simulink model "experiment_toplevel"  (R2016a)
settings: Solver=ode15s  StartTime=0.0  StopTime=20  MaxStep=1e-2  RelTol=1e-4
PreLoadFcn:
  | minitaurParameters
values from neighbouring files (symbols this model uses):
  angular_ctrl_d = 1    [minitaurParameters.m]
  angular_ctrl_i = 1    [minitaurParameters.m]
  angular_ctrl_p = 100    [minitaurParameters.m]
  enc_zero_IA = -1.25*pi    (= -3.92699081699)    [minitaurParameters.m]
  enc_zero_IB = -0.25*pi    (= -0.785398163397)    [minitaurParameters.m]
  enc_zero_IIA = 1.25*pi    (= 3.92699081699)    [minitaurParameters.m]
  enc_zero_IIB = 1.25*pi    (= 3.92699081699)    [minitaurParameters.m]
  enc_zero_IIIA = 0.5*pi    (= 1.57079632679)    [minitaurParameters.m]
  enc_zero_IIIB = 1.5*pi    (= 4.71238898038)    [minitaurParameters.m]
  enc_zero_IVA = -0.25*pi    (= -0.785398163397)    [minitaurParameters.m]
  enc_zero_IVB = 0.5*pi    (= 1.57079632679)    [minitaurParameters.m]
  fore_lag = fore_lag_vals(j)    [experiment1.m]    (also in experiment1_parfor_accelerator.m = 0; minitaurParameters.m = 0.45)
  ground_frame_depth = 0.5    [minitaurParameters.m]
  ground_length = 100    [minitaurParameters.m]
  ground_width = 10    [minitaurParameters.m]
  init_theta_IA = -pi/4    (= -0.785398163397)    [minitaurParameters.m]
  init_theta_IB = pi/4    (= 0.785398163397)    [minitaurParameters.m]
  init_theta_IIA = -pi/4    (= -0.785398163397)    [minitaurParameters.m]
  init_theta_IIB = pi/4    (= 0.785398163397)    [minitaurParameters.m]
  init_theta_IIIA = -pi/4    (= -0.785398163397)    [minitaurParameters.m]
  init_theta_IIIB = pi/4    (= 0.785398163397)    [minitaurParameters.m]
  init_theta_IVA = -pi/4    (= -0.785398163397)    [minitaurParameters.m]
  init_theta_IVB = pi/4    (= 0.785398163397)    [minitaurParameters.m]
  l1 = 100e-3    (= 0.1)    [minitaurParameters.m]
  l2 = 200e-3    (= 0.2)    [minitaurParameters.m]
  leg_joint_radius = 3e-3    (= 0.003)    [minitaurParameters.m]
  lr_sync = 1    [experiment1.m]    (also in experiment1_parfor_accelerator.m; minitaurParameters.m = 0)
  model = 'experiment_toplevel'    [experiment1_parfor_accelerator.m]
  period = period_vals(i)    [experiment1.m]    (also in experiment1_parfor_accelerator.m = 1.5; minitaurParameters.m = 0.33)
  phi_0 = 0.5*asin(l1/l2)    [experiment1.m]    (also in experiment1_parfor_accelerator.m; minitaurParameters.m)
  r_0 = l2    [experiment1.m]    (also in experiment1_parfor_accelerator.m; minitaurParameters.m = 0.2)
  r_x = 0.3*l1    [experiment1.m]    (also in experiment1_parfor_accelerator.m = 0.5*l1; minitaurParameters.m = 0.05)
  r_y = 0.2*l1    [experiment1.m]    (also in experiment1_parfor_accelerator.m = 0.3*l1; minitaurParameters.m = 0.03)
  radial_ctrl_d = 1    [minitaurParameters.m]
  radial_ctrl_i = 1    [minitaurParameters.m]
  radial_ctrl_p = 80    [minitaurParameters.m]
  safety_limit = 10e-3    (= 0.01)    [minitaurParameters.m]
undefined symbols (not defined in the file or in its folder): Axis, Fn, minitaurParams, r_stance, r_swing, stance_frac, X, Y, Z
undefined symbols (not defined in the file): leg_joint_fric_bw, leg_joint_mu_k, leg_joint_mu_s, leg_joint_vel_thresh, motor_kt, motor_kv, motor_r, motor_torque_sat
libraries: sm_lib x453, fl_lib x132, nesl_utility x31, Contact_Forces_Lib x28, simulink x19
(part 3 of 13)

== system experiment_toplevel/GR Minitaur/minitaur_leg_linkages_III ==
  Joint Friction Model : Subsystem  Variant=on  OverrideUsingVariant=stick-slip  mask(Joint Friction Model){modelVariant=Stick-Slip Friction, leg_joint_radius=leg_joint_radius, linear_region_thresh=leg_joint_vel_thresh, mu_k=leg_joint_mu_k, mu_s=leg_joint_mu_s, fric_bandwidth=leg_joint_fric_bw, mu_brk=0, fric_visc_coeff=0, trans_coeff=0}
      mask prompts: modelVariant "Friction Model"; leg_joint_radius "Leg Joint Effective Radius [m]"; linear_region_thresh "Linear Region Velocity Threshold [m/s]"; mu_k "Kinetic Friction Coefficient []"; mu_s "Static Friction Coefficient []"; fric_bandwidth "Friction Model Bandwidth [Hz]"; mu_brk "Breakaway Friction Coefficient []"; fric_visc_coeff "Viscous Friction Coefficient [N*s/m]"; trans_coeff "Transition Approximation Coefficient [s/m]"
      mask help: Models rotational friction present in passive joints. Two options available: stick-slip, and an advanced model that includes viscous and Stribeck friction. Note that in all models, friction is calculated as translational force couple, which is then converted to a friction torque (multiplied by effective joint diameter).
      mask TypeOptions modelVariant: Full Friction | Stick-Slip Friction
      mask Callback modelVariant:
      | currVariant = get_param(gcb,'modelVariant')
      | 
      | switch currVariant
      |     case 'Stick-Slip Friction'
      |         set_param(gcb,'OverrideUsingVariant','stick-slip')
      |         set_param(gcb,'MaskVisibilities',{'on';'on';'on';'on';'on';'on';'off';'off';'off'})
      |     case 'Full Friction'
      |         set_param(gcb,'OverrideUsingVariant','full')
      |         set_param(gcb,'MaskVisibilities',{'on';'on';'on';'on';'off';'off';'on';'on';'on'})
      | 
      | end
  Joint Friction Model1 : Subsystem  Variant=on  OverrideUsingVariant=stick-slip  mask(Joint Friction Model){modelVariant=Stick-Slip Friction, leg_joint_radius=leg_joint_radius, linear_region_thresh=leg_joint_vel_thresh, mu_k=leg_joint_mu_k, mu_s=leg_joint_mu_s, fric_bandwidth=leg_joint_fric_bw, mu_brk=0, fric_visc_coeff=0, trans_coeff=0}
      mask prompts: modelVariant "Friction Model"; leg_joint_radius "Leg Joint Effective Radius [m]"; linear_region_thresh "Linear Region Velocity Threshold [m/s]"; mu_k "Kinetic Friction Coefficient []"; mu_s "Static Friction Coefficient []"; fric_bandwidth "Friction Model Bandwidth [Hz]"; mu_brk "Breakaway Friction Coefficient []"; fric_visc_coeff "Viscous Friction Coefficient [N*s/m]"; trans_coeff "Transition Approximation Coefficient [s/m]"
      mask help: Models rotational friction present in passive joints. Two options available: stick-slip, and an advanced model that includes viscous and Stribeck friction. Note that in all models, friction is calculated as translational force couple, which is then converted to a friction torque (multiplied by effective joint diameter).
      mask TypeOptions modelVariant: Full Friction | Stick-Slip Friction
      mask Callback modelVariant:
      | currVariant = get_param(gcb,'modelVariant')
      | 
      | switch currVariant
      |     case 'Stick-Slip Friction'
      |         set_param(gcb,'OverrideUsingVariant','stick-slip')
      |         set_param(gcb,'MaskVisibilities',{'on';'on';'on';'on';'on';'on';'off';'off';'off'})
      |     case 'Full Friction'
      |         set_param(gcb,'OverrideUsingVariant','full')
      |         set_param(gcb,'MaskVisibilities',{'on';'on';'on';'on';'off';'off';'on';'on';'on'})
      | 
      | end
  Joint Friction Model2 : Subsystem  Variant=on  OverrideUsingVariant=stick-slip  mask(Joint Friction Model){modelVariant=Stick-Slip Friction, leg_joint_radius=leg_joint_radius, linear_region_thresh=leg_joint_vel_thresh, mu_k=leg_joint_mu_k, mu_s=leg_joint_mu_s, fric_bandwidth=leg_joint_fric_bw, mu_brk=0, fric_visc_coeff=0, trans_coeff=0}
      mask prompts: modelVariant "Friction Model"; leg_joint_radius "Leg Joint Effective Radius [m]"; linear_region_thresh "Linear Region Velocity Threshold [m/s]"; mu_k "Kinetic Friction Coefficient []"; mu_s "Static Friction Coefficient []"; fric_bandwidth "Friction Model Bandwidth [Hz]"; mu_brk "Breakaway Friction Coefficient []"; fric_visc_coeff "Viscous Friction Coefficient [N*s/m]"; trans_coeff "Transition Approximation Coefficient [s/m]"
      mask help: Models rotational friction present in passive joints. Two options available: stick-slip, and an advanced model that includes viscous and Stribeck friction. Note that in all models, friction is calculated as translational force couple, which is then converted to a friction torque (multiplied by effective joint diameter).
      mask TypeOptions modelVariant: Full Friction | Stick-Slip Friction
      mask Callback modelVariant:
      | currVariant = get_param(gcb,'modelVariant')
      | 
      | switch currVariant
      |     case 'Stick-Slip Friction'
      |         set_param(gcb,'OverrideUsingVariant','stick-slip')
      |         set_param(gcb,'MaskVisibilities',{'on';'on';'on';'on';'on';'on';'off';'off';'off'})
      |     case 'Full Friction'
      |         set_param(gcb,'OverrideUsingVariant','full')
      |         set_param(gcb,'MaskVisibilities',{'on';'on';'on';'on';'off';'off';'on';'on';'on'})
      | 
      | end
  ReferenceFrame : sm_lib/Frames and Transforms/Reference Frame
  Revolute : sm_lib/Joints/Revolute Joint  SenseConstraintForce=off  SenseConstraintForceX=off  SenseConstraintForceY=off  SenseConstraintForceZ=off  SenseConstraintTorque=off  SenseConstraintTorqueX=off  SenseConstraintTorqueY=off  SenseConstraintTorqueZ=off  SenseTotalForce=on  SenseTotalForceX=off  SenseTotalForceY=off  SenseTotalForceZ=off  SenseTotalTorque=off  SenseTotalTorqueX=off  SenseTotalTorqueY=off  SenseTotalTorqueZ=off  CompositeWrenchDir=FollowerOnBase  CompositeWrenchFrame=BaseFrame  EquilibriumPosition=0  EquilibriumPositionUnits=rad  SpringStiffness=0  SpringStiffnessUnits=m*N/rad  DampingCoefficient=0  DampingCoefficientUnits=m*s*N/rad  TorqueActuationMode=InputTorque  MotionActuationMode=ComputedMotion  SensePosition=off  SenseVelocity=on  SenseAcceleration=off  SenseTorqueForce=off  PositionTargetSpecify=off  PositionTargetPriority=Low  PositionTargetValue=minitaurParams.RevoluteJoint(1).Rz.Pos  PositionTargetValueUnits=deg  VelocityTargetSpecify=off  VelocityTargetPriority=High  VelocityTargetValue=0  VelocityTargetValueUnits=deg/s
  Revolute1 : sm_lib/Joints/Revolute Joint  SenseConstraintForce=off  SenseConstraintForceX=off  SenseConstraintForceY=off  SenseConstraintForceZ=off  SenseConstraintTorque=off  SenseConstraintTorqueX=off  SenseConstraintTorqueY=off  SenseConstraintTorqueZ=off  SenseTotalForce=on  SenseTotalForceX=off  SenseTotalForceY=off  SenseTotalForceZ=off  SenseTotalTorque=off  SenseTotalTorqueX=off  SenseTotalTorqueY=off  SenseTotalTorqueZ=off  CompositeWrenchDir=FollowerOnBase  CompositeWrenchFrame=BaseFrame  EquilibriumPosition=0  EquilibriumPositionUnits=rad  SpringStiffness=0  SpringStiffnessUnits=m*N/rad  DampingCoefficient=0  DampingCoefficientUnits=m*s*N/rad  TorqueActuationMode=InputTorque  MotionActuationMode=ComputedMotion  SensePosition=off  SenseVelocity=on  SenseAcceleration=off  SenseTorqueForce=off  PositionTargetSpecify=on  PositionTargetPriority=Low  PositionTargetValue=init_toe_joint_l  PositionTargetValueUnits=rad  VelocityTargetSpecify=off  VelocityTargetPriority=High  VelocityTargetValue=0  VelocityTargetValueUnits=deg/s
  Revolute2 : sm_lib/Joints/Revolute Joint  SenseConstraintForce=off  SenseConstraintForceX=off  SenseConstraintForceY=off  SenseConstraintForceZ=off  SenseConstraintTorque=off  SenseConstraintTorqueX=off  SenseConstraintTorqueY=off  SenseConstraintTorqueZ=off  SenseTotalForce=on  SenseTotalForceX=off  SenseTotalForceY=off  SenseTotalForceZ=off  SenseTotalTorque=off  SenseTotalTorqueX=off  SenseTotalTorqueY=off  SenseTotalTorqueZ=off  CompositeWrenchDir=FollowerOnBase  CompositeWrenchFrame=BaseFrame  EquilibriumPosition=0  EquilibriumPositionUnits=rad  SpringStiffness=0  SpringStiffnessUnits=m*N/rad  DampingCoefficient=0  DampingCoefficientUnits=m*s*N/rad  TorqueActuationMode=InputTorque  MotionActuationMode=ComputedMotion  SensePosition=off  SenseVelocity=on  SenseAcceleration=off  SenseTorqueForce=off  PositionTargetSpecify=off  PositionTargetPriority=Low  PositionTargetValue=minitaurParams.RevoluteJoint(3).Rz.Pos  PositionTargetValueUnits=deg  VelocityTargetSpecify=off  VelocityTargetPriority=High  VelocityTargetValue=0  VelocityTargetValueUnits=deg/s
  Transform : sm_lib/Frames and Transforms/Rigid Transform  TranslationMethod=Cartesian  TranslationLengthUnit=mm  TranslationStandardAxis=+Z  TranslationStandardOffset=0  TranslationCartesianOffset=minitaurParams.RigidTransform(16).translation  TranslationROffset=0  TranslationROffsetUnits=m  TranslationZOffset=0  TranslationZOffsetUnits=m  TranslationThetaOffset=0  TranslationThetaOffsetUnits=deg  RotationMethod=ArbitraryAxis  RotationAngleUnits=rad  RotationStandardAxis=+Z  RotationAngle=minitaurParams.RigidTransform(16).angle  RotationArbitraryAxis=minitaurParams.RigidTransform(16).axis  FollAlignAxisA=+X  BaseAlignAxisA=+Y  FollAlignAxisB=+Y  BaseAlignAxisB=+Z  RotationSequenceAxes=FollowerAxes  RotationSequence=XYX  RotationSequenceAngles=[0 0 0]  RotationSequenceAnglesUnits=deg  RotationMatrix=[1 0 0; 0 1 0; 0 0 1]
  minitaur_leg_joint_placeholder_sim_1_RIGID : Subsystem
  minitaur_leg_joint_placeholder_sim_2_RIGID : Subsystem
  minitaur_leg_joint_placeholder_sim_3_RIGID : Subsystem
  minitaur_leg_lower_link_1_RIGID : Subsystem
  minitaur_leg_lower_link_toe_1_RIGID : Subsystem
  minitaur_leg_upper_link_2_RIGID : Subsystem
  minitaur_leg_upper_link_3_RIGID : Subsystem
  x2517T32_2_RIGID : Subsystem
  F1 : PMIOPort  Port=1  Side=Left
  F : PMIOPort  Port=2  Side=Left
  F_contact : PMIOPort  Port=3  Side=Right
  connections:
  minitaur_leg_upper_link_3_RIGID/RConn1 -- Revolute/LConn1
  ReferenceFrame/RConn1 -- Transform/LConn1
  Transform/RConn1 -- minitaur_leg_upper_link_2_RIGID/LConn1
  minitaur_leg_upper_link_2_RIGID/LConn2 -- F/RConn1
  minitaur_leg_upper_link_3_RIGID/LConn1 -- F1/RConn1
  minitaur_leg_lower_link_toe_1_RIGID/RConn2 -- Revolute1/LConn1
  minitaur_leg_joint_placeholder_sim_2_RIGID/LConn1 -- minitaur_leg_lower_link_toe_1_RIGID/LConn2
  Revolute2/LConn1 -- minitaur_leg_lower_link_toe_1_RIGID/RConn1
  x2517T32_2_RIGID/LConn1 -- minitaur_leg_lower_link_toe_1_RIGID/LConn1
  minitaur_leg_joint_placeholder_sim_1_RIGID/LConn1 -- minitaur_leg_upper_link_3_RIGID/LConn2
  minitaur_leg_joint_placeholder_sim_3_RIGID/LConn1 -- minitaur_leg_upper_link_2_RIGID/LConn4
  F_contact/RConn1 -- x2517T32_2_RIGID/RConn1
  Joint Friction Model2/RConn1 -- Revolute/LConn2
  Joint Friction Model1/RConn1 -- Revolute1/LConn2
  Revolute/RConn1 -- minitaur_leg_lower_link_1_RIGID/LConn2
  Revolute2/LConn2 -- Joint Friction Model/RConn1
  Revolute2/RConn1 -- minitaur_leg_upper_link_2_RIGID/LConn3
  Revolute2/RConn3 -- Joint Friction Model/LConn2
  Joint Friction Model1/LConn2 -- Revolute1/RConn3
  Revolute/RConn2 -- Joint Friction Model2/LConn1
  Revolute2/RConn2 -- Joint Friction Model/LConn1
  Revolute/RConn3 -- Joint Friction Model2/LConn2
  Revolute1/RConn2 -- Joint Friction Model1/LConn1
  Revolute1/RConn1 -- minitaur_leg_lower_link_1_RIGID/LConn1

== system experiment_toplevel/GR Minitaur/minitaur_leg_linkages_IV ==
  Joint Friction Model : Subsystem  Variant=on  OverrideUsingVariant=stick-slip  mask(Joint Friction Model){modelVariant=Stick-Slip Friction, leg_joint_radius=leg_joint_radius, linear_region_thresh=leg_joint_vel_thresh, mu_k=leg_joint_mu_k, mu_s=leg_joint_mu_s, fric_bandwidth=leg_joint_fric_bw, mu_brk=0, fric_visc_coeff=0, trans_coeff=0}
      mask prompts: modelVariant "Friction Model"; leg_joint_radius "Leg Joint Effective Radius [m]"; linear_region_thresh "Linear Region Velocity Threshold [m/s]"; mu_k "Kinetic Friction Coefficient []"; mu_s "Static Friction Coefficient []"; fric_bandwidth "Friction Model Bandwidth [Hz]"; mu_brk "Breakaway Friction Coefficient []"; fric_visc_coeff "Viscous Friction Coefficient [N*s/m]"; trans_coeff "Transition Approximation Coefficient [s/m]"
      mask help: Models rotational friction present in passive joints. Two options available: stick-slip, and an advanced model that includes viscous and Stribeck friction. Note that in all models, friction is calculated as translational force couple, which is then converted to a friction torque (multiplied by effective joint diameter).
      mask TypeOptions modelVariant: Full Friction | Stick-Slip Friction
      mask Callback modelVariant:
      | currVariant = get_param(gcb,'modelVariant')
      | 
      | switch currVariant
      |     case 'Stick-Slip Friction'
      |         set_param(gcb,'OverrideUsingVariant','stick-slip')
      |         set_param(gcb,'MaskVisibilities',{'on';'on';'on';'on';'on';'on';'off';'off';'off'})
      |     case 'Full Friction'
      |         set_param(gcb,'OverrideUsingVariant','full')
      |         set_param(gcb,'MaskVisibilities',{'on';'on';'on';'on';'off';'off';'on';'on';'on'})
      | 
      | end
  Joint Friction Model1 : Subsystem  Variant=on  OverrideUsingVariant=stick-slip  mask(Joint Friction Model){modelVariant=Stick-Slip Friction, leg_joint_radius=leg_joint_radius, linear_region_thresh=leg_joint_vel_thresh, mu_k=leg_joint_mu_k, mu_s=leg_joint_mu_s, fric_bandwidth=leg_joint_fric_bw, mu_brk=0, fric_visc_coeff=0, trans_coeff=0}
      mask prompts: modelVariant "Friction Model"; leg_joint_radius "Leg Joint Effective Radius [m]"; linear_region_thresh "Linear Region Velocity Threshold [m/s]"; mu_k "Kinetic Friction Coefficient []"; mu_s "Static Friction Coefficient []"; fric_bandwidth "Friction Model Bandwidth [Hz]"; mu_brk "Breakaway Friction Coefficient []"; fric_visc_coeff "Viscous Friction Coefficient [N*s/m]"; trans_coeff "Transition Approximation Coefficient [s/m]"
      mask help: Models rotational friction present in passive joints. Two options available: stick-slip, and an advanced model that includes viscous and Stribeck friction. Note that in all models, friction is calculated as translational force couple, which is then converted to a friction torque (multiplied by effective joint diameter).
      mask TypeOptions modelVariant: Full Friction | Stick-Slip Friction
      mask Callback modelVariant:
      | currVariant = get_param(gcb,'modelVariant')
      | 
      | switch currVariant
      |     case 'Stick-Slip Friction'
      |         set_param(gcb,'OverrideUsingVariant','stick-slip')
      |         set_param(gcb,'MaskVisibilities',{'on';'on';'on';'on';'on';'on';'off';'off';'off'})
      |     case 'Full Friction'
      |         set_param(gcb,'OverrideUsingVariant','full')
      |         set_param(gcb,'MaskVisibilities',{'on';'on';'on';'on';'off';'off';'on';'on';'on'})
      | 
      | end
  Joint Friction Model2 : Subsystem  Variant=on  OverrideUsingVariant=stick-slip  mask(Joint Friction Model){modelVariant=Stick-Slip Friction, leg_joint_radius=leg_joint_radius, linear_region_thresh=leg_joint_vel_thresh, mu_k=leg_joint_mu_k, mu_s=leg_joint_mu_s, fric_bandwidth=leg_joint_fric_bw, mu_brk=0, fric_visc_coeff=0, trans_coeff=0}
      mask prompts: modelVariant "Friction Model"; leg_joint_radius "Leg Joint Effective Radius [m]"; linear_region_thresh "Linear Region Velocity Threshold [m/s]"; mu_k "Kinetic Friction Coefficient []"; mu_s "Static Friction Coefficient []"; fric_bandwidth "Friction Model Bandwidth [Hz]"; mu_brk "Breakaway Friction Coefficient []"; fric_visc_coeff "Viscous Friction Coefficient [N*s/m]"; trans_coeff "Transition Approximation Coefficient [s/m]"
      mask help: Models rotational friction present in passive joints. Two options available: stick-slip, and an advanced model that includes viscous and Stribeck friction. Note that in all models, friction is calculated as translational force couple, which is then converted to a friction torque (multiplied by effective joint diameter).
      mask TypeOptions modelVariant: Full Friction | Stick-Slip Friction
      mask Callback modelVariant:
      | currVariant = get_param(gcb,'modelVariant')
      | 
      | switch currVariant
      |     case 'Stick-Slip Friction'
      |         set_param(gcb,'OverrideUsingVariant','stick-slip')
      |         set_param(gcb,'MaskVisibilities',{'on';'on';'on';'on';'on';'on';'off';'off';'off'})
      |     case 'Full Friction'
      |         set_param(gcb,'OverrideUsingVariant','full')
      |         set_param(gcb,'MaskVisibilities',{'on';'on';'on';'on';'off';'off';'on';'on';'on'})
      | 
      | end
  ReferenceFrame : sm_lib/Frames and Transforms/Reference Frame
  Revolute : sm_lib/Joints/Revolute Joint  SenseConstraintForce=off  SenseConstraintForceX=off  SenseConstraintForceY=off  SenseConstraintForceZ=off  SenseConstraintTorque=off  SenseConstraintTorqueX=off  SenseConstraintTorqueY=off  SenseConstraintTorqueZ=off  SenseTotalForce=on  SenseTotalForceX=off  SenseTotalForceY=off  SenseTotalForceZ=off  SenseTotalTorque=off  SenseTotalTorqueX=off  SenseTotalTorqueY=off  SenseTotalTorqueZ=off  CompositeWrenchDir=FollowerOnBase  CompositeWrenchFrame=BaseFrame  EquilibriumPosition=0  EquilibriumPositionUnits=rad  SpringStiffness=0  SpringStiffnessUnits=m*N/rad  DampingCoefficient=0  DampingCoefficientUnits=m*s*N/rad  TorqueActuationMode=InputTorque  MotionActuationMode=ComputedMotion  SensePosition=off  SenseVelocity=on  SenseAcceleration=off  SenseTorqueForce=off  PositionTargetSpecify=off  PositionTargetPriority=Low  PositionTargetValue=minitaurParams.RevoluteJoint(1).Rz.Pos  PositionTargetValueUnits=deg  VelocityTargetSpecify=off  VelocityTargetPriority=High  VelocityTargetValue=0  VelocityTargetValueUnits=deg/s
  Revolute1 : sm_lib/Joints/Revolute Joint  SenseConstraintForce=off  SenseConstraintForceX=off  SenseConstraintForceY=off  SenseConstraintForceZ=off  SenseConstraintTorque=off  SenseConstraintTorqueX=off  SenseConstraintTorqueY=off  SenseConstraintTorqueZ=off  SenseTotalForce=on  SenseTotalForceX=off  SenseTotalForceY=off  SenseTotalForceZ=off  SenseTotalTorque=off  SenseTotalTorqueX=off  SenseTotalTorqueY=off  SenseTotalTorqueZ=off  CompositeWrenchDir=FollowerOnBase  CompositeWrenchFrame=BaseFrame  EquilibriumPosition=0  EquilibriumPositionUnits=rad  SpringStiffness=0  SpringStiffnessUnits=m*N/rad  DampingCoefficient=0  DampingCoefficientUnits=m*s*N/rad  TorqueActuationMode=InputTorque  MotionActuationMode=ComputedMotion  SensePosition=off  SenseVelocity=on  SenseAcceleration=off  SenseTorqueForce=off  PositionTargetSpecify=on  PositionTargetPriority=Low  PositionTargetValue=init_toe_joint_r  PositionTargetValueUnits=rad  VelocityTargetSpecify=off  VelocityTargetPriority=High  VelocityTargetValue=0  VelocityTargetValueUnits=deg/s
  Revolute2 : sm_lib/Joints/Revolute Joint  SenseConstraintForce=off  SenseConstraintForceX=off  SenseConstraintForceY=off  SenseConstraintForceZ=off  SenseConstraintTorque=off  SenseConstraintTorqueX=off  SenseConstraintTorqueY=off  SenseConstraintTorqueZ=off  SenseTotalForce=on  SenseTotalForceX=off  SenseTotalForceY=off  SenseTotalForceZ=off  SenseTotalTorque=off  SenseTotalTorqueX=off  SenseTotalTorqueY=off  SenseTotalTorqueZ=off  CompositeWrenchDir=FollowerOnBase  CompositeWrenchFrame=BaseFrame  EquilibriumPosition=0  EquilibriumPositionUnits=rad  SpringStiffness=0  SpringStiffnessUnits=m*N/rad  DampingCoefficient=0  DampingCoefficientUnits=m*s*N/rad  TorqueActuationMode=InputTorque  MotionActuationMode=ComputedMotion  SensePosition=off  SenseVelocity=on  SenseAcceleration=off  SenseTorqueForce=off  PositionTargetSpecify=off  PositionTargetPriority=Low  PositionTargetValue=minitaurParams.RevoluteJoint(3).Rz.Pos  PositionTargetValueUnits=deg  VelocityTargetSpecify=off  VelocityTargetPriority=High  VelocityTargetValue=0  VelocityTargetValueUnits=deg/s
  Transform : sm_lib/Frames and Transforms/Rigid Transform  TranslationMethod=Cartesian  TranslationLengthUnit=mm  TranslationStandardAxis=+Z  TranslationStandardOffset=0  TranslationCartesianOffset=minitaurParams.RigidTransform(16).translation  TranslationROffset=0  TranslationROffsetUnits=m  TranslationZOffset=0  TranslationZOffsetUnits=m  TranslationThetaOffset=0  TranslationThetaOffsetUnits=deg  RotationMethod=ArbitraryAxis  RotationAngleUnits=rad  RotationStandardAxis=+Z  RotationAngle=minitaurParams.RigidTransform(16).angle  RotationArbitraryAxis=minitaurParams.RigidTransform(16).axis  FollAlignAxisA=+X  BaseAlignAxisA=+Y  FollAlignAxisB=+Y  BaseAlignAxisB=+Z  RotationSequenceAxes=FollowerAxes  RotationSequence=XYX  RotationSequenceAngles=[0 0 0]  RotationSequenceAnglesUnits=deg  RotationMatrix=[1 0 0; 0 1 0; 0 0 1]
  minitaur_leg_joint_placeholder_sim_1_RIGID : Subsystem
  minitaur_leg_joint_placeholder_sim_2_RIGID : Subsystem
  minitaur_leg_joint_placeholder_sim_3_RIGID : Subsystem
  minitaur_leg_lower_link_1_RIGID : Subsystem
  minitaur_leg_lower_link_toe_1_RIGID : Subsystem
  minitaur_leg_upper_link_2_RIGID : Subsystem
  minitaur_leg_upper_link_3_RIGID : Subsystem
  x2517T32_2_RIGID : Subsystem
  F : PMIOPort  Port=1  Side=Left
  F1 : PMIOPort  Port=2  Side=Left
  F_contact : PMIOPort  Port=3  Side=Right
  connections:
  ReferenceFrame/RConn1 -- Transform/LConn1
  Transform/RConn1 -- minitaur_leg_upper_link_2_RIGID/LConn1
  minitaur_leg_upper_link_3_RIGID/LConn1 -- F/RConn1
  minitaur_leg_upper_link_2_RIGID/LConn2 -- F1/RConn1
  minitaur_leg_joint_placeholder_sim_2_RIGID/LConn1 -- minitaur_leg_lower_link_toe_1_RIGID/LConn2
  x2517T32_2_RIGID/LConn1 -- minitaur_leg_lower_link_toe_1_RIGID/LConn1
  minitaur_leg_joint_placeholder_sim_1_RIGID/LConn1 -- minitaur_leg_upper_link_3_RIGID/LConn2
  minitaur_leg_joint_placeholder_sim_3_RIGID/LConn1 -- minitaur_leg_upper_link_2_RIGID/LConn4
  F_contact/RConn1 -- x2517T32_2_RIGID/RConn1
  Joint Friction Model2/RConn1 -- Revolute/LConn2
  Joint Friction Model1/RConn1 -- Revolute1/LConn2
  Revolute/RConn1 -- minitaur_leg_lower_link_1_RIGID/LConn2
  Joint Friction Model/RConn1 -- Revolute2/LConn2
  Revolute2/RConn1 -- minitaur_leg_upper_link_2_RIGID/LConn3
  Joint Friction Model/LConn2 -- Revolute2/RConn3
  Joint Friction Model1/LConn2 -- Revolute1/RConn3
  Revolute/RConn2 -- Joint Friction Model2/LConn1
  Joint Friction Model/LConn1 -- Revolute2/RConn2
  Revolute/RConn3 -- Joint Friction Model2/LConn2
  Revolute1/RConn2 -- Joint Friction Model1/LConn1
  minitaur_leg_lower_link_toe_1_RIGID/RConn1 -- Revolute2/LConn1
  minitaur_leg_lower_link_toe_1_RIGID/RConn2 -- Revolute1/LConn1
  minitaur_leg_upper_link_3_RIGID/RConn1 -- Revolute/LConn1
  minitaur_leg_lower_link_1_RIGID/LConn1 -- Revolute1/RConn1

== system experiment_toplevel/GR Minitaur/minitaur_motor_module_IA ==
  Desired Torque : Inport
  DYS_BLDC_86x10_BE8108_12 : Subsystem
  Encoder Model : Subsystem  mask{enc_zero=enc_zero_IA}
      mask prompts: enc_zero "Encoder Zero Value [rad]"
  ReferenceFrame : sm_lib/Frames and Transforms/Reference Frame
  Transform : sm_lib/Frames and Transforms/Rigid Transform  TranslationMethod=Cartesian  TranslationLengthUnit=mm  TranslationStandardAxis=+Z  TranslationStandardOffset=0  TranslationCartesianOffset=minitaurParams.RigidTransform(24).translation  TranslationROffset=0  TranslationROffsetUnits=m  TranslationZOffset=0  TranslationZOffsetUnits=m  TranslationThetaOffset=0  TranslationThetaOffsetUnits=deg  RotationMethod=ArbitraryAxis  RotationAngleUnits=rad  RotationStandardAxis=+Z  RotationAngle=minitaurParams.RigidTransform(24).angle  RotationArbitraryAxis=minitaurParams.RigidTransform(24).axis  FollAlignAxisA=+X  BaseAlignAxisA=+Y  FollAlignAxisB=+Y  BaseAlignAxisB=+Z  RotationSequenceAxes=FollowerAxes  RotationSequence=XYX  RotationSequenceAngles=[0 0 0]  RotationSequenceAnglesUnits=deg  RotationMatrix=[1 0 0; 0 1 0; 0 0 1]
  minitaur_motor_driver_board_1_RIGID : Subsystem
  minitaur_motor_driver_cover_1_RIGID : Subsystem
  minitaur_motor_module_plate_1_RIGID : Subsystem
  F1 : PMIOPort  Port=1  Side=Left
  F : PMIOPort  Port=2  Side=Left
  Encoder Value : Outport
  Mech Power : Outport  Port=2
  Input Power : Outport  Port=3
  wires:
  Encoder Model/1(Encoder Value) -> Encoder Value/1
  DYS_BLDC_86x10_BE8108_12/1(Mech Power) -> Mech Power/1
  Desired Torque/1 -> DYS_BLDC_86x10_BE8108_12/1(Desired Torque)
  DYS_BLDC_86x10_BE8108_12/2(Position) -> Encoder Model/1(Motor Position)
  DYS_BLDC_86x10_BE8108_12/3(Input Power) -> Input Power/1
  connections:
  minitaur_motor_driver_cover_1_RIGID/LConn2 -- minitaur_motor_module_plate_1_RIGID/LConn1
  ReferenceFrame/RConn1 -- Transform/LConn1
  Transform/RConn1 -- minitaur_motor_module_plate_1_RIGID/LConn2
  minitaur_motor_module_plate_1_RIGID/LConn3 -- DYS_BLDC_86x10_BE8108_12/LConn1
  minitaur_motor_driver_board_1_RIGID/LConn1 -- minitaur_motor_driver_cover_1_RIGID/LConn1
  DYS_BLDC_86x10_BE8108_12/LConn2 -- F/RConn1
  DYS_BLDC_86x10_BE8108_12/LConn3 -- F1/RConn1

== system experiment_toplevel/GR Minitaur/minitaur_motor_module_IB ==
  Desired Torque : Inport
  DYS_BLDC_86x10_BE8108_12 : Subsystem
  Encoder Model : Subsystem  mask{enc_zero=enc_zero_IB}
      mask prompts: enc_zero "Encoder Zero Value [rad]"
  ReferenceFrame : sm_lib/Frames and Transforms/Reference Frame
  Transform : sm_lib/Frames and Transforms/Rigid Transform  TranslationMethod=Cartesian  TranslationLengthUnit=mm  TranslationStandardAxis=+Z  TranslationStandardOffset=0  TranslationCartesianOffset=minitaurParams.RigidTransform(24).translation  TranslationROffset=0  TranslationROffsetUnits=m  TranslationZOffset=0  TranslationZOffsetUnits=m  TranslationThetaOffset=0  TranslationThetaOffsetUnits=deg  RotationMethod=ArbitraryAxis  RotationAngleUnits=rad  RotationStandardAxis=+Z  RotationAngle=minitaurParams.RigidTransform(24).angle  RotationArbitraryAxis=minitaurParams.RigidTransform(24).axis  FollAlignAxisA=+X  BaseAlignAxisA=+Y  FollAlignAxisB=+Y  BaseAlignAxisB=+Z  RotationSequenceAxes=FollowerAxes  RotationSequence=XYX  RotationSequenceAngles=[0 0 0]  RotationSequenceAnglesUnits=deg  RotationMatrix=[1 0 0; 0 1 0; 0 0 1]
  minitaur_motor_driver_board_1_RIGID : Subsystem
  minitaur_motor_driver_cover_1_RIGID : Subsystem
  minitaur_motor_module_plate_1_RIGID : Subsystem
  F1 : PMIOPort  Port=1  Side=Left
  F : PMIOPort  Port=2  Side=Left
  Encoder Value : Outport
  Mech Power : Outport  Port=2
  Input Power : Outport  Port=3
  wires:
  Encoder Model/1(Encoder Value) -> Encoder Value/1
  DYS_BLDC_86x10_BE8108_12/1(Mech Power) -> Mech Power/1
  DYS_BLDC_86x10_BE8108_12/2(Position) -> Encoder Model/1(Motor Position)
  Desired Torque/1 -> DYS_BLDC_86x10_BE8108_12/1(Desired Torque)
  DYS_BLDC_86x10_BE8108_12/3(Input Power) -> Input Power/1
  connections:
  minitaur_motor_driver_cover_1_RIGID/LConn2 -- minitaur_motor_module_plate_1_RIGID/LConn1
  ReferenceFrame/RConn1 -- Transform/LConn1
  Transform/RConn1 -- minitaur_motor_module_plate_1_RIGID/LConn2
  DYS_BLDC_86x10_BE8108_12/LConn1 -- minitaur_motor_module_plate_1_RIGID/LConn3
  minitaur_motor_driver_board_1_RIGID/LConn1 -- minitaur_motor_driver_cover_1_RIGID/LConn1
  DYS_BLDC_86x10_BE8108_12/LConn2 -- F/RConn1
  DYS_BLDC_86x10_BE8108_12/LConn3 -- F1/RConn1

== system experiment_toplevel/GR Minitaur/minitaur_motor_module_IIA ==
  Desired Torque : Inport
  DYS_BLDC_86x10_BE8108_12 : Subsystem
  Encoder Model : Subsystem  mask{enc_zero=enc_zero_IIA}
      mask prompts: enc_zero "Encoder Zero Value [rad]"
  ReferenceFrame : sm_lib/Frames and Transforms/Reference Frame
  Transform : sm_lib/Frames and Transforms/Rigid Transform  TranslationMethod=Cartesian  TranslationLengthUnit=mm  TranslationStandardAxis=+Z  TranslationStandardOffset=0  TranslationCartesianOffset=minitaurParams.RigidTransform(24).translation  TranslationROffset=0  TranslationROffsetUnits=m  TranslationZOffset=0  TranslationZOffsetUnits=m  TranslationThetaOffset=0  TranslationThetaOffsetUnits=deg  RotationMethod=ArbitraryAxis  RotationAngleUnits=rad  RotationStandardAxis=+Z  RotationAngle=minitaurParams.RigidTransform(24).angle  RotationArbitraryAxis=minitaurParams.RigidTransform(24).axis  FollAlignAxisA=+X  BaseAlignAxisA=+Y  FollAlignAxisB=+Y  BaseAlignAxisB=+Z  RotationSequenceAxes=FollowerAxes  RotationSequence=XYX  RotationSequenceAngles=[0 0 0]  RotationSequenceAnglesUnits=deg  RotationMatrix=[1 0 0; 0 1 0; 0 0 1]
  minitaur_motor_driver_board_1_RIGID : Subsystem
  minitaur_motor_driver_cover_1_RIGID : Subsystem
  minitaur_motor_module_plate_1_RIGID : Subsystem
  F1 : PMIOPort  Port=1  Side=Left
  F : PMIOPort  Port=2  Side=Left
  Encoder Value : Outport
  Mech Power : Outport  Port=2
  Input Power : Outport  Port=3
  wires:
  Encoder Model/1(Encoder Value) -> Encoder Value/1
  Desired Torque/1 -> DYS_BLDC_86x10_BE8108_12/1(Desired Torque)
  DYS_BLDC_86x10_BE8108_12/3(Input Power) -> Input Power/1
  DYS_BLDC_86x10_BE8108_12/2(Position) -> Encoder Model/1(Motor Position)
  DYS_BLDC_86x10_BE8108_12/1(Mech Power) -> Mech Power/1
  connections:
  minitaur_motor_driver_cover_1_RIGID/LConn2 -- minitaur_motor_module_plate_1_RIGID/LConn1
  ReferenceFrame/RConn1 -- Transform/LConn1
  Transform/RConn1 -- minitaur_motor_module_plate_1_RIGID/LConn2
  DYS_BLDC_86x10_BE8108_12/LConn1 -- minitaur_motor_module_plate_1_RIGID/LConn3
  minitaur_motor_driver_board_1_RIGID/LConn1 -- minitaur_motor_driver_cover_1_RIGID/LConn1
  DYS_BLDC_86x10_BE8108_12/LConn2 -- F/RConn1
  DYS_BLDC_86x10_BE8108_12/LConn3 -- F1/RConn1

== system experiment_toplevel/GR Minitaur/minitaur_motor_module_IIB ==
  Desired Torque : Inport
  DYS_BLDC_86x10_BE8108_12 : Subsystem
  Encoder Model : Subsystem  mask{enc_zero=enc_zero_IIB}
      mask prompts: enc_zero "Encoder Zero Value [rad]"
  ReferenceFrame : sm_lib/Frames and Transforms/Reference Frame
  Transform : sm_lib/Frames and Transforms/Rigid Transform  TranslationMethod=Cartesian  TranslationLengthUnit=mm  TranslationStandardAxis=+Z  TranslationStandardOffset=0  TranslationCartesianOffset=minitaurParams.RigidTransform(24).translation  TranslationROffset=0  TranslationROffsetUnits=m  TranslationZOffset=0  TranslationZOffsetUnits=m  TranslationThetaOffset=0  TranslationThetaOffsetUnits=deg  RotationMethod=ArbitraryAxis  RotationAngleUnits=rad  RotationStandardAxis=+Z  RotationAngle=minitaurParams.RigidTransform(24).angle  RotationArbitraryAxis=minitaurParams.RigidTransform(24).axis  FollAlignAxisA=+X  BaseAlignAxisA=+Y  FollAlignAxisB=+Y  BaseAlignAxisB=+Z  RotationSequenceAxes=FollowerAxes  RotationSequence=XYX  RotationSequenceAngles=[0 0 0]  RotationSequenceAnglesUnits=deg  RotationMatrix=[1 0 0; 0 1 0; 0 0 1]
  minitaur_motor_driver_board_1_RIGID : Subsystem
  minitaur_motor_driver_cover_1_RIGID : Subsystem
  minitaur_motor_module_plate_1_RIGID : Subsystem
  F1 : PMIOPort  Port=1  Side=Left
  F : PMIOPort  Port=2  Side=Left
  Encoder Value : Outport
  Mech Power : Outport  Port=2
  Input Power : Outport  Port=3
  wires:
  Encoder Model/1(Encoder Value) -> Encoder Value/1
  DYS_BLDC_86x10_BE8108_12/1(Mech Power) -> Mech Power/1
  DYS_BLDC_86x10_BE8108_12/2(Position) -> Encoder Model/1(Motor Position)
  Desired Torque/1 -> DYS_BLDC_86x10_BE8108_12/1(Desired Torque)
  DYS_BLDC_86x10_BE8108_12/3(Input Power) -> Input Power/1
  connections:
  minitaur_motor_driver_cover_1_RIGID/LConn2 -- minitaur_motor_module_plate_1_RIGID/LConn1
  ReferenceFrame/RConn1 -- Transform/LConn1
  Transform/RConn1 -- minitaur_motor_module_plate_1_RIGID/LConn2
  DYS_BLDC_86x10_BE8108_12/LConn1 -- minitaur_motor_module_plate_1_RIGID/LConn3
  minitaur_motor_driver_board_1_RIGID/LConn1 -- minitaur_motor_driver_cover_1_RIGID/LConn1
  DYS_BLDC_86x10_BE8108_12/LConn2 -- F/RConn1
  DYS_BLDC_86x10_BE8108_12/LConn3 -- F1/RConn1

== system experiment_toplevel/GR Minitaur/minitaur_motor_module_IIIA ==
  Desired Torque : Inport
  DYS_BLDC_86x10_BE8108_12 : Subsystem
  Encoder Model : Subsystem  mask{enc_zero=enc_zero_IIIA}
      mask prompts: enc_zero "Encoder Zero Value [rad]"
  ReferenceFrame : sm_lib/Frames and Transforms/Reference Frame
  Transform : sm_lib/Frames and Transforms/Rigid Transform  TranslationMethod=Cartesian  TranslationLengthUnit=mm  TranslationStandardAxis=+Z  TranslationStandardOffset=0  TranslationCartesianOffset=minitaurParams.RigidTransform(24).translation  TranslationROffset=0  TranslationROffsetUnits=m  TranslationZOffset=0  TranslationZOffsetUnits=m  TranslationThetaOffset=0  TranslationThetaOffsetUnits=deg  RotationMethod=ArbitraryAxis  RotationAngleUnits=rad  RotationStandardAxis=+Z  RotationAngle=minitaurParams.RigidTransform(24).angle  RotationArbitraryAxis=minitaurParams.RigidTransform(24).axis  FollAlignAxisA=+X  BaseAlignAxisA=+Y  FollAlignAxisB=+Y  BaseAlignAxisB=+Z  RotationSequenceAxes=FollowerAxes  RotationSequence=XYX  RotationSequenceAngles=[0 0 0]  RotationSequenceAnglesUnits=deg  RotationMatrix=[1 0 0; 0 1 0; 0 0 1]
  minitaur_motor_driver_board_1_RIGID : Subsystem
  minitaur_motor_driver_cover_1_RIGID : Subsystem
  minitaur_motor_module_plate_1_RIGID : Subsystem
  F : PMIOPort  Port=1  Side=Left
  F1 : PMIOPort  Port=2  Side=Left
  Encoder Value : Outport
  Mech Power : Outport  Port=2
  Input Power : Outport  Port=3
  wires:
  Encoder Model/1(Encoder Value) -> Encoder Value/1
  DYS_BLDC_86x10_BE8108_12/1(Mech Power) -> Mech Power/1
  DYS_BLDC_86x10_BE8108_12/2(Position) -> Encoder Model/1(Motor Position)
  Desired Torque/1 -> DYS_BLDC_86x10_BE8108_12/1(Desired Torque)
  DYS_BLDC_86x10_BE8108_12/3(Input Power) -> Input Power/1
  connections:
  minitaur_motor_driver_cover_1_RIGID/LConn2 -- minitaur_motor_module_plate_1_RIGID/LConn1
  ReferenceFrame/RConn1 -- Transform/LConn1
  Transform/RConn1 -- minitaur_motor_module_plate_1_RIGID/LConn2
  DYS_BLDC_86x10_BE8108_12/LConn1 -- minitaur_motor_module_plate_1_RIGID/LConn3
  minitaur_motor_driver_board_1_RIGID/LConn1 -- minitaur_motor_driver_cover_1_RIGID/LConn1
  DYS_BLDC_86x10_BE8108_12/LConn2 -- F/RConn1
  DYS_BLDC_86x10_BE8108_12/LConn3 -- F1/RConn1

== system experiment_toplevel/GR Minitaur/minitaur_motor_module_IIIB ==
  Desired Torque : Inport
  DYS_BLDC_86x10_BE8108_12 : Subsystem
  Encoder Model : Subsystem  mask{enc_zero=enc_zero_IIIB}
      mask prompts: enc_zero "Encoder Zero Value [rad]"
  ReferenceFrame : sm_lib/Frames and Transforms/Reference Frame
  Transform : sm_lib/Frames and Transforms/Rigid Transform  TranslationMethod=Cartesian  TranslationLengthUnit=mm  TranslationStandardAxis=+Z  TranslationStandardOffset=0  TranslationCartesianOffset=minitaurParams.RigidTransform(24).translation  TranslationROffset=0  TranslationROffsetUnits=m  TranslationZOffset=0  TranslationZOffsetUnits=m  TranslationThetaOffset=0  TranslationThetaOffsetUnits=deg  RotationMethod=ArbitraryAxis  RotationAngleUnits=rad  RotationStandardAxis=+Z  RotationAngle=minitaurParams.RigidTransform(24).angle  RotationArbitraryAxis=minitaurParams.RigidTransform(24).axis  FollAlignAxisA=+X  BaseAlignAxisA=+Y  FollAlignAxisB=+Y  BaseAlignAxisB=+Z  RotationSequenceAxes=FollowerAxes  RotationSequence=XYX  RotationSequenceAngles=[0 0 0]  RotationSequenceAnglesUnits=deg  RotationMatrix=[1 0 0; 0 1 0; 0 0 1]
  minitaur_motor_driver_board_1_RIGID : Subsystem
  minitaur_motor_driver_cover_1_RIGID : Subsystem
  minitaur_motor_module_plate_1_RIGID : Subsystem
  F1 : PMIOPort  Port=1  Side=Left
  F : PMIOPort  Port=2  Side=Left
  Encoder Value : Outport
  Mech Power : Outport  Port=2
  Input Power : Outport  Port=3
  wires:
  Encoder Model/1(Encoder Value) -> Encoder Value/1
  Desired Torque/1 -> DYS_BLDC_86x10_BE8108_12/1(Desired Torque)
  DYS_BLDC_86x10_BE8108_12/3(Input Power) -> Input Power/1
  DYS_BLDC_86x10_BE8108_12/2(Position) -> Encoder Model/1(Motor Position)
  DYS_BLDC_86x10_BE8108_12/1(Mech Power) -> Mech Power/1
  connections:
  minitaur_motor_driver_cover_1_RIGID/LConn2 -- minitaur_motor_module_plate_1_RIGID/LConn1
  ReferenceFrame/RConn1 -- Transform/LConn1
  Transform/RConn1 -- minitaur_motor_module_plate_1_RIGID/LConn2
  DYS_BLDC_86x10_BE8108_12/LConn1 -- minitaur_motor_module_plate_1_RIGID/LConn3
  minitaur_motor_driver_board_1_RIGID/LConn1 -- minitaur_motor_driver_cover_1_RIGID/LConn1
  DYS_BLDC_86x10_BE8108_12/LConn2 -- F/RConn1
  DYS_BLDC_86x10_BE8108_12/LConn3 -- F1/RConn1

== system experiment_toplevel/GR Minitaur/minitaur_motor_module_IVA ==
  Desired Torque : Inport
  DYS_BLDC_86x10_BE8108_12 : Subsystem
  Encoder Model : Subsystem  mask{enc_zero=enc_zero_IVA}
      mask prompts: enc_zero "Encoder Zero Value [rad]"
  ReferenceFrame : sm_lib/Frames and Transforms/Reference Frame
  Transform : sm_lib/Frames and Transforms/Rigid Transform  TranslationMethod=Cartesian  TranslationLengthUnit=mm  TranslationStandardAxis=+Z  TranslationStandardOffset=0  TranslationCartesianOffset=minitaurParams.RigidTransform(24).translation  TranslationROffset=0  TranslationROffsetUnits=m  TranslationZOffset=0  TranslationZOffsetUnits=m  TranslationThetaOffset=0  TranslationThetaOffsetUnits=deg  RotationMethod=ArbitraryAxis  RotationAngleUnits=rad  RotationStandardAxis=+Z  RotationAngle=minitaurParams.RigidTransform(24).angle  RotationArbitraryAxis=minitaurParams.RigidTransform(24).axis  FollAlignAxisA=+X  BaseAlignAxisA=+Y  FollAlignAxisB=+Y  BaseAlignAxisB=+Z  RotationSequenceAxes=FollowerAxes  RotationSequence=XYX  RotationSequenceAngles=[0 0 0]  RotationSequenceAnglesUnits=deg  RotationMatrix=[1 0 0; 0 1 0; 0 0 1]
  minitaur_motor_driver_board_1_RIGID : Subsystem
  minitaur_motor_driver_cover_1_RIGID : Subsystem
  minitaur_motor_module_plate_1_RIGID : Subsystem
  F : PMIOPort  Port=1  Side=Left
  F1 : PMIOPort  Port=2  Side=Left
  Encoder Value : Outport
  Mech Power : Outport  Port=2
  Input Power : Outport  Port=3
  wires:
  Encoder Model/1(Encoder Value) -> Encoder Value/1
  DYS_BLDC_86x10_BE8108_12/1(Mech Power) -> Mech Power/1
  DYS_BLDC_86x10_BE8108_12/2(Position) -> Encoder Model/1(Motor Position)
  Desired Torque/1 -> DYS_BLDC_86x10_BE8108_12/1(Voltage)
  DYS_BLDC_86x10_BE8108_12/3(Input Power) -> Input Power/1
  connections:
  minitaur_motor_driver_cover_1_RIGID/LConn2 -- minitaur_motor_module_plate_1_RIGID/LConn1
  ReferenceFrame/RConn1 -- Transform/LConn1
  Transform/RConn1 -- minitaur_motor_module_plate_1_RIGID/LConn2
  DYS_BLDC_86x10_BE8108_12/LConn1 -- minitaur_motor_module_plate_1_RIGID/LConn3
  minitaur_motor_driver_board_1_RIGID/LConn1 -- minitaur_motor_driver_cover_1_RIGID/LConn1
  DYS_BLDC_86x10_BE8108_12/LConn2 -- F/RConn1
  DYS_BLDC_86x10_BE8108_12/LConn3 -- F1/RConn1

== system experiment_toplevel/GR Minitaur/minitaur_motor_module_IVB ==
  Desired Torque : Inport
  DYS_BLDC_86x10_BE8108_12 : Subsystem
  Encoder Model : Subsystem  mask{enc_zero=enc_zero_IVB}
      mask prompts: enc_zero "Encoder Zero Value [rad]"
  ReferenceFrame : sm_lib/Frames and Transforms/Reference Frame
  Transform : sm_lib/Frames and Transforms/Rigid Transform  TranslationMethod=Cartesian  TranslationLengthUnit=mm  TranslationStandardAxis=+Z  TranslationStandardOffset=0  TranslationCartesianOffset=minitaurParams.RigidTransform(24).translation  TranslationROffset=0  TranslationROffsetUnits=m  TranslationZOffset=0  TranslationZOffsetUnits=m  TranslationThetaOffset=0  TranslationThetaOffsetUnits=deg  RotationMethod=ArbitraryAxis  RotationAngleUnits=rad  RotationStandardAxis=+Z  RotationAngle=minitaurParams.RigidTransform(24).angle  RotationArbitraryAxis=minitaurParams.RigidTransform(24).axis  FollAlignAxisA=+X  BaseAlignAxisA=+Y  FollAlignAxisB=+Y  BaseAlignAxisB=+Z  RotationSequenceAxes=FollowerAxes  RotationSequence=XYX  RotationSequenceAngles=[0 0 0]  RotationSequenceAnglesUnits=deg  RotationMatrix=[1 0 0; 0 1 0; 0 0 1]
  minitaur_motor_driver_board_1_RIGID : Subsystem
  minitaur_motor_driver_cover_1_RIGID : Subsystem
  minitaur_motor_module_plate_1_RIGID : Subsystem
  F1 : PMIOPort  Port=1  Side=Left
  F : PMIOPort  Port=2  Side=Left
  Encoder Value : Outport
  Mech Power : Outport  Port=2
  Input Power : Outport  Port=3
  wires:
  Encoder Model/1(Encoder Value) -> Encoder Value/1
  Desired Torque/1 -> DYS_BLDC_86x10_BE8108_12/1(Voltage)
  DYS_BLDC_86x10_BE8108_12/1(Mech Power) -> Mech Power/1
  DYS_BLDC_86x10_BE8108_12/2(Position) -> Encoder Model/1(Motor Position)
  DYS_BLDC_86x10_BE8108_12/3(Input Power) -> Input Power/1
  connections:
  minitaur_motor_driver_cover_1_RIGID/LConn2 -- minitaur_motor_module_plate_1_RIGID/LConn1
  ReferenceFrame/RConn1 -- Transform/LConn1
  Transform/RConn1 -- minitaur_motor_module_plate_1_RIGID/LConn2
  DYS_BLDC_86x10_BE8108_12/LConn1 -- minitaur_motor_module_plate_1_RIGID/LConn3
  minitaur_motor_driver_board_1_RIGID/LConn1 -- minitaur_motor_driver_cover_1_RIGID/LConn1
  DYS_BLDC_86x10_BE8108_12/LConn2 -- F/RConn1
  DYS_BLDC_86x10_BE8108_12/LConn3 -- F1/RConn1

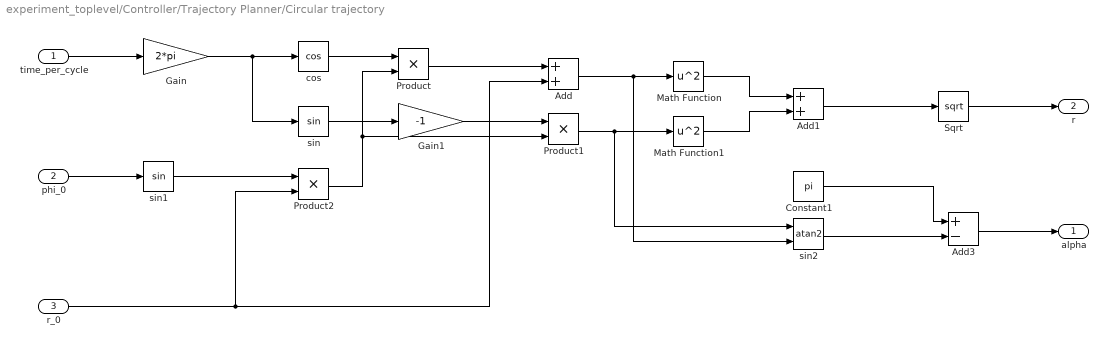
== system experiment_toplevel/Controller/Trajectory Planner/Circular trajectory ==
  time_per_cycle : Inport
  phi_0 : Inport  Port=2
  r_0 : Inport  Port=3
  Add : Sum
  Add1 : Sum
  Add3 : Sum  Inputs=+-
  Constant1 : Constant  Value=pi
  Gain : Gain  Gain=2*pi
  Gain1 : Gain  Gain=-1
  Math Function : Math  Operator=square  SaturateOnIntegerOverflow=on
  Math Function1 : Math  Operator=square  SaturateOnIntegerOverflow=on
  Product : Product
  Product1 : Product
  Product2 : Product
  Sqrt : Sqrt  SaturateOnIntegerOverflow=on
  cos : Trigonometry  Operator=cos
  sin : Trigonometry
  sin1 : Trigonometry
  sin2 : Trigonometry  Operator=atan2
  alpha : Outport
  r : Outport  Port=2
  wires:
  time_per_cycle/1 -> Gain/1
  Gain/1 -> sin/1, cos/1
  cos/1 -> Product/1
  phi_0/1 -> sin1/1
  sin1/1 -> Product2/1
  r_0/1 -> Add/2, Product2/2
  Product2/1 -> Product1/2, Product/2
  Add/1 -> sin2/2, Math Function/1
  Product1/1 -> sin2/1, Math Function1/1
  Math Function/1 -> Add1/1
  Math Function1/1 -> Add1/2
  Sqrt/1 -> r/1
  Add1/1 -> Sqrt/1
  Constant1/1 -> Add3/1
  sin2/1 -> Add3/2
  Add3/1 -> alpha/1
  sin/1 -> Gain1/1
  Product/1 -> Add/1
  Gain1/1 -> Product1/1

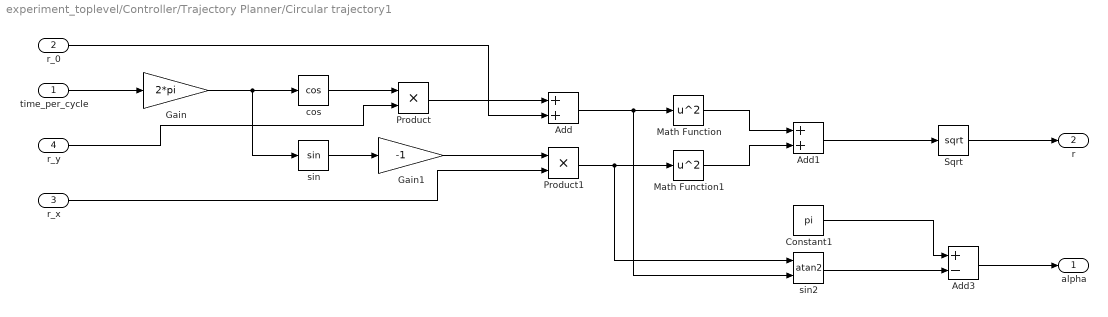
== system experiment_toplevel/Controller/Trajectory Planner/Circular trajectory1 ==
  time_per_cycle : Inport
  r_0 : Inport  Port=2
  r_x : Inport  Port=3
  r_y : Inport  Port=4
  Add : Sum
  Add1 : Sum
  Add3 : Sum  Inputs=+-
  Constant1 : Constant  Value=pi
  Gain : Gain  Gain=2*pi
  Gain1 : Gain  Gain=-1
  Math Function : Math  Operator=square  SaturateOnIntegerOverflow=on
  Math Function1 : Math  Operator=square  SaturateOnIntegerOverflow=on
  Product : Product
  Product1 : Product
  Sqrt : Sqrt  SaturateOnIntegerOverflow=on
  cos : Trigonometry  Operator=cos
  sin : Trigonometry
  sin2 : Trigonometry  Operator=atan2
  alpha : Outport
  r : Outport  Port=2
  wires:
  Product/1 -> Add/1
  sin/1 -> Gain1/1
  Add3/1 -> alpha/1
  sin2/1 -> Add3/2
  Constant1/1 -> Add3/1
  Add1/1 -> Sqrt/1
  Sqrt/1 -> r/1
  Math Function1/1 -> Add1/2
  Math Function/1 -> Add1/1
  Product1/1 -> Math Function1/1, sin2/1
  Add/1 -> Math Function/1, sin2/2
  r_0/1 -> Add/2
  cos/1 -> Product/1
  Gain/1 -> cos/1, sin/1
  time_per_cycle/1 -> Gain/1
  r_y/1 -> Product/2
  r_x/1 -> Product1/2
  Gain1/1 -> Product1/1

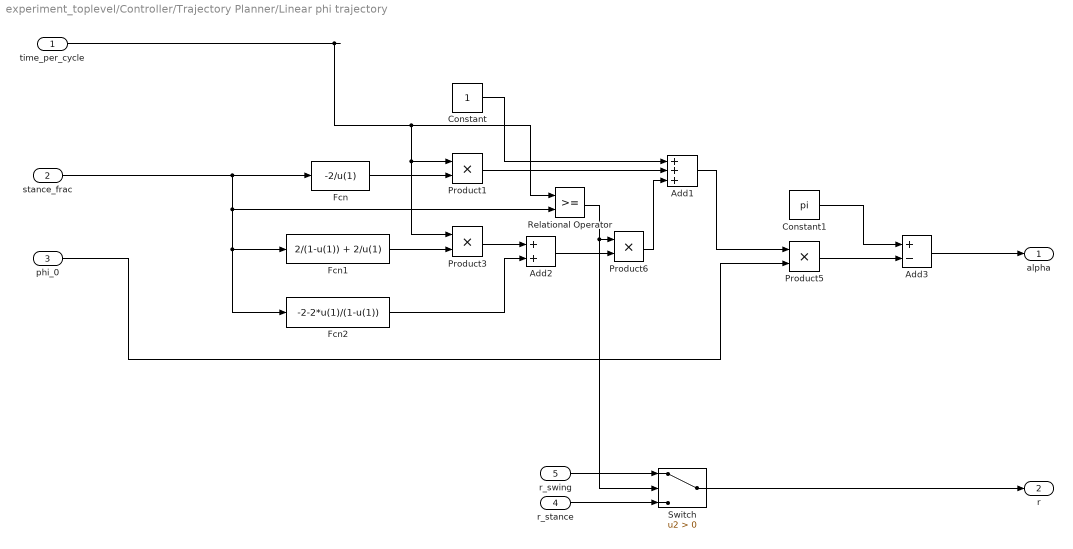
== system experiment_toplevel/Controller/Trajectory Planner/Linear phi trajectory ==
  time_per_cycle : Inport
  stance_frac : Inport  Port=2
  phi_0 : Inport  Port=3
  "r_stance " : Inport  Port=4
  r_swing : Inport  Port=5
  Add1 : Sum  Inputs=+++
  Add2 : Sum
  Add3 : Sum  Inputs=+-
  Constant : Constant
  Constant1 : Constant  Value=pi
  Fcn : Fcn  Expr=-2/u(1)
  Fcn1 : Fcn  Expr=2/(1-u(1)) + 2/u(1)
  Fcn2 : Fcn  Expr=-2-2*u(1)/(1-u(1))
  Product{1,3,5..6} (4 alike) : Product
  Relational Operator : RelationalOperator  OutDataTypeStr=boolean
  Switch : Switch  Criteria=u2 > Threshold
  alpha : Outport
  r : Outport  Port=2
  wires:
  Add2/1 -> Product6/2
  phi_0/1 -> Product5/2
  Fcn/1 -> Product1/2
  Product5/1 -> Add3/2
  Relational Operator/1 -> Switch/2, Product6/1
  Add3/1 -> alpha/1
  stance_frac/1 -> Fcn1/1, Fcn2/1, Relational Operator/2, Fcn/1
  Product6/1 -> Add1/3
  Add1/1 -> Product5/1
  Product1/1 -> Add1/2
  Fcn1/1 -> Product3/2
  Constant/1 -> Add1/1
  time_per_cycle/1 -> Relational Operator/1, Product1/1, Product3/1
  Fcn2/1 -> Add2/2
  Product3/1 -> Add2/1
  Constant1/1 -> Add3/1
  r_swing/1 -> Switch/1
  "r_stance "/1 -> Switch/3
  Switch/1 -> r/1

== system experiment_toplevel/Controller/Trajectory Planner/Phase offset ==
  note: Legs:
      | Right Fore
      | Left Fore
      | Left Rear
      | Right Rear
  note: Boolean: left/right in sync (true) or
      | 180* out of phase(false)
  note: Fraction of period that a fore leg
      | lags behind its corresponding rear leg
  fore_lag_in : Inport
  lr_sync : Inport  Port=2
  Add : Sum
  Constant : Constant  Value=[0.5 0 0 0.5]
  Constant1 : Constant  Value=[0 0 1 1]
  Logical Operator : Logic  Operator=NOT  AllPortsSameDT=off  OutDataTypeStr=boolean
  Product : Product
  Product1 : Product
  phase offsets : Outport
  wires:
  fore_lag_in/1 -> Product/1
  Constant1/1 -> Product/2
  lr_sync/1 -> Logical Operator/1
  Constant/1 -> Product1/2
  Product/1 -> Add/1
  Product1/1 -> Add/2
  Add/1 -> phase offsets/1
  Logical Operator/1 -> Product1/1

== system experiment_toplevel/Controller/Trajectory Planner/Rerouter  ==
  alpha : Inport
  r : Inport  Port=2
  Demux : Demux
  Demux1 : Demux
  Mux{,1..3} (4 alike) : Mux  Inputs=2
  leg 1 : Outport
  leg 2 : Outport  Port=2
  leg 3 : Outport  Port=3
  leg 4 : Outport  Port=4
  wires:
  Demux1/1 -> Mux/2
  Mux1/1 -> leg 2/1
  Demux/2 -> Mux1/1
  Demux/1 -> Mux/1
  alpha/1 -> Demux/1
  Mux/1 -> leg 1/1
  Demux1/2 -> Mux1/2
  Mux3/1 -> leg 4/1
  Demux/4 -> Mux3/1
  Mux2/1 -> leg 3/1
  r/1 -> Demux1/1
  Demux/3 -> Mux2/1
  Demux1/3 -> Mux2/2
  Demux1/4 -> Mux3/2

== system experiment_toplevel/Controller/Trajectory Planner/Rerouter 1 ==
  alpha : Inport
  r : Inport  Port=2
  Demux : Demux
  Demux1 : Demux
  Mux{,1..3} (4 alike) : Mux  Inputs=2
  leg 1 : Outport
  leg 2 : Outport  Port=2
  leg 3 : Outport  Port=3
  leg 4 : Outport  Port=4
  wires:
  Demux1/4 -> Mux3/2
  Demux1/3 -> Mux2/2
  Demux/3 -> Mux2/1
  r/1 -> Demux1/1
  Mux2/1 -> leg 3/1
  Demux/4 -> Mux3/1
  Mux3/1 -> leg 4/1
  Demux1/2 -> Mux1/2
  Mux/1 -> leg 1/1
  alpha/1 -> Demux/1
  Demux/1 -> Mux/1
  Demux/2 -> Mux1/1
  Mux1/1 -> leg 2/1
  Demux1/1 -> Mux/2
